simulink model "LQR_observer"  (R2022b)
settings: Solver=ode45  StartTime=0.0  StopTime=simulation_time  MaxStep=0.01  RelTol=1e-3  EnableMultiTasking=on
values from neighbouring files (symbols this model uses):
  AObs = [Phi - L*Cprime]    [ex2.m]
  BObs = [Gam L]    [ex2.m]
  C = eye(5)    [ex1.m]    (also in exercise2_LQRandObserver.m = Corig)
  CObs = eye(size(Phi))    [ex2.m]
  Cprim = [1 0 0 0 0 ... (first row only)    [ex2.m]
  DObs = zeros(size(Phi,1), size(L,2) + size(Gam,2))    [ex2.m]
  parameters = sol1.getSystemParameters    [exercise2_LQRandObserver.m]
  path_to_track =     [path_4.mat]
  sampling_time = 0.01    [exercise2_LQRandObserver.m]
  x0 = {x0_experiment_1}    [ex1.m]
  x0Obs = [0.01, 0, -0.02, 0, 0]    [ex2.m]
undefined symbols (not defined in the file or in its folder): lqr_gain, LQR_input_signal_ID
settings Model: Creator=ezequiel  LastModifiedBy=bapti
settings SolverCC: AlgebraicLoopSolver=TrustRegion
settings DataIOCC: ReturnWorkspaceOutputs=off
settings OptimizationCC: LifeSpan=inf
settings DebuggingCC: UnconnectedInputMsg=warning  UnconnectedOutputMsg=warning  UnconnectedLineMsg=warning  AllowSymbolicDim=off  PregeneratedLibrarySubsystemCodeDiagnostic=none  SFUnexpectedBacktrackingDiag=warning  SFNoUnconditionalDefaultTransitionDiag=warning  SFExecutionAtInitializationDiag=none  SFMachineParentedDataDiag=warning  ArithmeticOperatorsInVariantConditions=warning
settings ModelReferenceCC: EnableRefExpFcnMdlSchedulingChecks=on  PropagateSignalLabelsOutOfModel=off
settings SFSimCC: SimUseLocalCustomCode=off  CustomCodeUndefinedFunction=UseInterfaceOnly
settings RTWCC: RTWUseLocalCustomCode=off
settings CodeAppCC: StateflowObjectComments=on
settings GRTTargetCC: TargetLangStandard=C89/C90 (ANSI)
settings ConfigComp: CovMetricSettings=dw  CovSaveCumulativeToWorkspaceVar=on  CovSaveSingleToWorkspaceVar=on  CovExternalEMLEnable=off

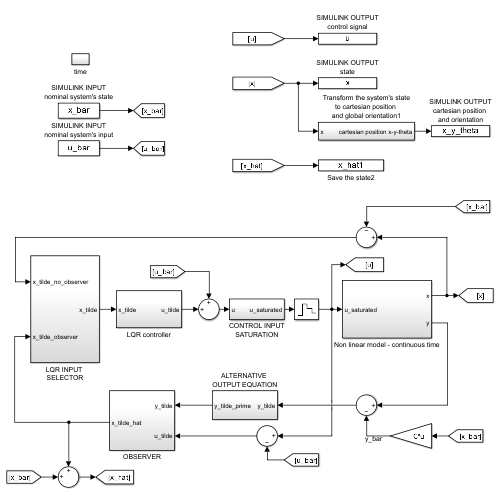
[thumbnail: Simulink's stored preview of the top-level diagram]
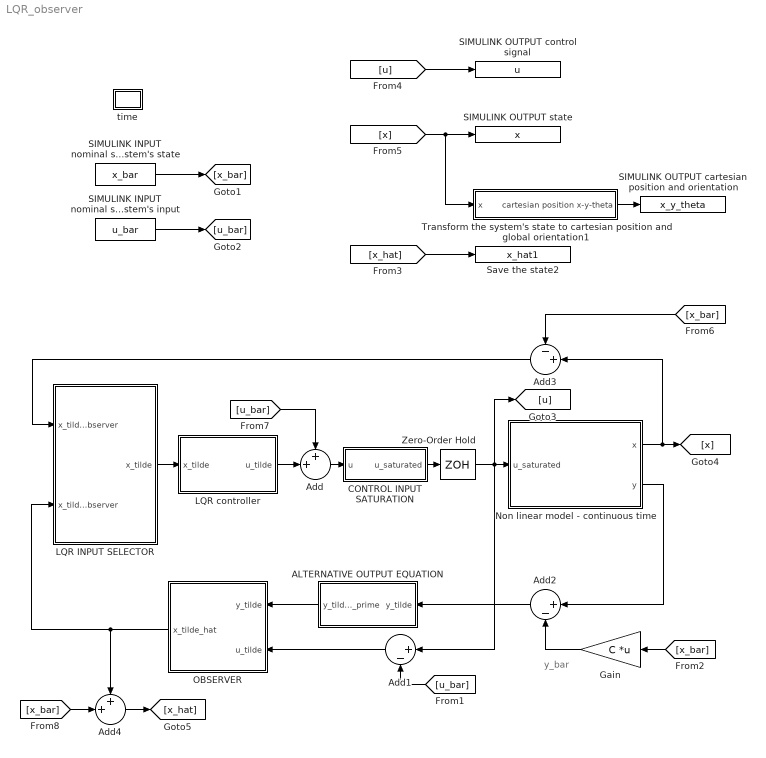
== system LQR_observer ==
  note: y_bar
  ALTERNATIVE OUTPUT EQUATION : Subsystem
  Add : Sum  Inputs=++|
  Add1 : Sum  Inputs=|+-
  Add2 : Sum  Inputs=|+-
  Add3 : Sum  Inputs=-+|
  Add4 : Sum  Inputs=++|
  CONTROL INPUT SATURATION : Subsystem
  Gain : Gain  Gain=C  Multiplication=Matrix(K*u)
  LQR INPUT SELECTOR : Subsystem
  LQR controller : Subsystem
  Non linear model - continuous time : Subsystem
  OBSERVER : Subsystem
  SIMULINK INPUT nominal system's input : FromWorkspace  VariableName=u_bar  SampleTime=sampling_time  OutputAfterFinalValue=Holding final value
  SIMULINK INPUT nominal system's state : FromWorkspace  VariableName=x_bar  SampleTime=sampling_time  OutputAfterFinalValue=Holding final value
  SIMULINK OUTPUT cartesian position and orientation : ToWorkspace  VariableName=x_y_theta  SampleTime=-1
  SIMULINK OUTPUT control signal : ToWorkspace  VariableName=u  SampleTime=-1
  SIMULINK OUTPUT state : ToWorkspace  VariableName=x  SampleTime=-1
  Save the state2 : ToWorkspace  VariableName=x_hat1  SampleTime=-1
  Transform the system's state to cartesian position and global orientation1 : Subsystem
  Zero-Order Hold : ZeroOrderHold  SampleTime=sampling_time
  time : Subsystem
  wires:
  SIMULINK INPUT nominal system's state/1 -> [x_bar]
  SIMULINK INPUT nominal system's input/1 -> [u_bar]
  [u] -> SIMULINK OUTPUT control signal/1
  [x] -> Transform the system's state to cartesian position and global orientation1/1(x), SIMULINK OUTPUT state/1
  Transform the system's state to cartesian position and global orientation1/1(cartesian position x-y-theta) -> SIMULINK OUTPUT cartesian position and orientation/1
  LQR INPUT SELECTOR/1(x_tilde) -> LQR controller/1(x_tilde)
  LQR controller/1(u_tilde) -> Add/2
  Add/1 -> CONTROL INPUT SATURATION/1(u)
  [u_bar] -> Add/1
  ALTERNATIVE OUTPUT EQUATION/1(y_tilde_prime) -> OBSERVER/1(y_tilde)
  OBSERVER/1(x_tilde_hat) -> LQR INPUT SELECTOR/2(x_tilde_observer), Add4/1
  [u_bar] -> Add1/2
  Add1/1 -> OBSERVER/2(u_tilde)
  [x_bar] -> Gain/1
  Gain/1 -> Add2/2
  Non linear model - continuous time/2(y) -> Add2/1
  Add2/1 -> ALTERNATIVE OUTPUT EQUATION/1(y_tilde)
  Non linear model - continuous time/1(x) -> [x], Add3/2
  Add3/1 -> LQR INPUT SELECTOR/1("x_tilde_no_observer ")
  [x_hat] -> Save the state2/1
  [x_bar] -> Add4/2
  Add4/1 -> [x_hat]
  [x_bar] -> Add3/1
  CONTROL INPUT SATURATION/1(u_saturated) -> Zero-Order Hold/1
  Zero-Order Hold/1 -> Add1/1, [u], Non linear model - continuous time/1(u_saturated)

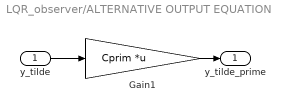
== system LQR_observer/ALTERNATIVE OUTPUT EQUATION ==
  y_tilde : Inport
  Gain1 : Gain  Gain=Cprim  Multiplication=Matrix(K*u)
  y_tilde_prime : Outport  VectorParamsAs1DForOutWhenUnconnected=off
  wires:
  Gain1/1 -> y_tilde_prime/1
  y_tilde/1 -> Gain1/1

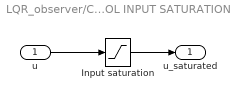
== system LQR_observer/CONTROL INPUT SATURATION ==
  u : Inport
  Input saturation : Saturate  UpperLimit=[Inf;4*pi]  LowerLimit=[0;-4*pi]
  u_saturated : Outport  VectorParamsAs1DForOutWhenUnconnected=off
  wires:
  u/1 -> Input saturation/1
  Input saturation/1 -> u_saturated/1

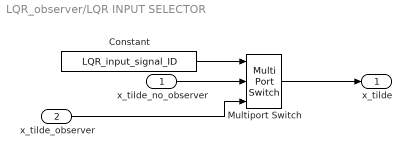
== system LQR_observer/LQR INPUT SELECTOR ==
  "x_tilde_no_observer " : Inport  PortDimensions=5
  x_tilde_observer : Inport  Port=2  PortDimensions=5
  Constant : Constant  Value=LQR_input_signal_ID
  Multiport Switch : MultiPortSwitch  Inputs=2  SaturateOnIntegerOverflow=off  InputSameDT=off
  x_tilde : Outport  VectorParamsAs1DForOutWhenUnconnected=off
  wires:
  "x_tilde_no_observer "/1 -> Multiport Switch/2
  x_tilde_observer/1 -> Multiport Switch/3
  Constant/1 -> Multiport Switch/1
  Multiport Switch/1 -> x_tilde/1

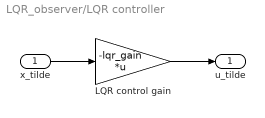
== system LQR_observer/LQR controller ==
  x_tilde : Inport  PortDimensions=5
  LQR control gain : Gain  Gain=-lqr_gain  Multiplication=Matrix(K*u)
  u_tilde : Outport  VectorParamsAs1DForOutWhenUnconnected=off
  wires:
  x_tilde/1 -> LQR control gain/1
  LQR control gain/1 -> u_tilde/1

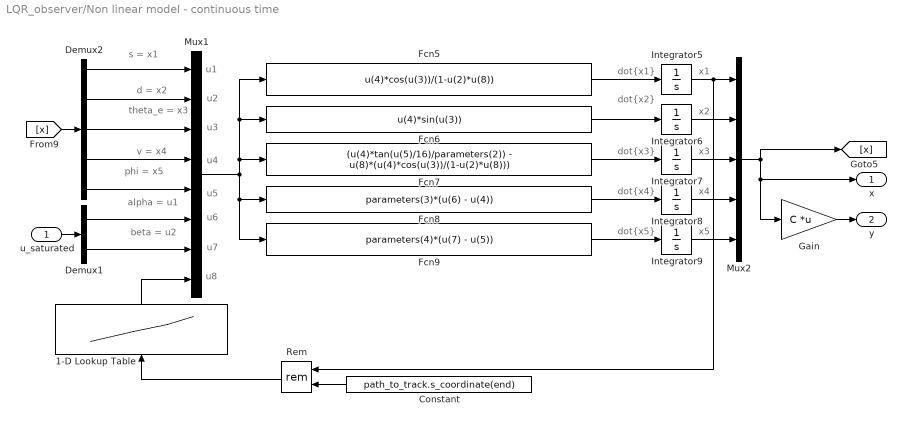
== system LQR_observer/Non linear model - continuous time ==
  note: s = x1
  note: dot{x1}
  note: d = x2
  note: theta_e = x3
  note: v = x4
  note: phi = x5
  note: alpha = u1
  note: beta = u2
  note: u1
  note: u2
  note: u3
  note: u4
  note: u5
  note: u6
  note: u7
  note: x1
  note: dot{x2}
  note: x2
  note: dot{x3}
  note: x3
  note: dot{x4}
  note: x4
  note: dot{x5}
  note: x5
  note: u8
  u_saturated : Inport
  1-D Lookup Table : Lookup_n-D  NumberOfTableDimensions=1  BreakpointsForDimension1=path_to_track.s_coordinate  Table=path_to_track.curvature  InternalRulePriority=Speed  RndMeth=Simplest
  Constant : Constant  Value=path_to_track.s_coordinate(end)
  Demux1 : Demux  Outputs=2
  Demux2 : Demux  Outputs=5
  Fcn5 : Fcn  Expr=u(4)*cos(u(3))/(1-u(2)*u(8))
  Fcn6 : Fcn  Expr=u(4)*sin(u(3))
  Fcn7 : Fcn  Expr=(u(4)*tan(u(5)/16)/parameters(2)) - u(8)*(u(4)*cos(u(3))/(1-u(2)*u(8)))
  Fcn8 : Fcn  Expr=parameters(3)*(u(6) - u(4))
  Fcn9 : Fcn  Expr=parameters(4)*(u(7) - u(5))
  Gain : Gain  Gain=C  Multiplication=Matrix(K*u)
  Integrator5 : Integrator  InitialCondition=x0(1)
  Integrator6 : Integrator  InitialCondition=x0(2)
  Integrator7 : Integrator  InitialCondition=x0(3)
  Integrator8 : Integrator  InitialCondition=x0(4)
  Integrator9 : Integrator  InitialCondition=x0(5)
  Mux1 : Mux  Inputs=8
  Mux2 : Mux  Inputs=5
  Rem : Math  Operator=rem  SignedPower=on
  x : Outport  VectorParamsAs1DForOutWhenUnconnected=off
  y : Outport  Port=2  VectorParamsAs1DForOutWhenUnconnected=off
  wires:
  u_saturated/1 -> Demux1/1
  Demux2/1 -> Mux1/1
  Demux2/2 -> Mux1/2
  Demux2/3 -> Mux1/3
  Demux2/4 -> Mux1/4
  Demux2/5 -> Mux1/5
  Demux1/1 -> Mux1/6
  Demux1/2 -> Mux1/7
  Integrator6/1 -> Mux2/2
  Integrator7/1 -> Mux2/3
  Integrator8/1 -> Mux2/4
  Integrator9/1 -> Mux2/5
  [x] -> Demux2/1
  1-D Lookup Table/1 -> Mux1/8
  Rem/1 -> 1-D Lookup Table/1
  Constant/1 -> Rem/2
  Integrator5/1 -> Rem/1, Mux2/1
  Mux2/1 -> Gain/1, x/1, [x]
  Gain/1 -> y/1
  Mux1/1 -> Fcn6/1, Fcn5/1, Fcn7/1, Fcn9/1, Fcn8/1
  Fcn8/1 -> Integrator8/1
  Fcn9/1 -> Integrator9/1
  Fcn7/1 -> Integrator7/1
  Fcn5/1 -> Integrator5/1
  Fcn6/1 -> Integrator6/1

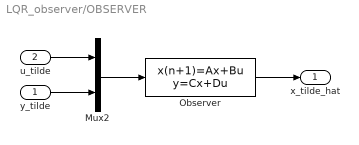
== system LQR_observer/OBSERVER ==
  y_tilde : Inport
  u_tilde : Inport  Port=2
  Mux2 : Mux  Inputs=2
  Observer : DiscreteStateSpace  A=AObs  B=BObs  C=CObs  D=DObs  InitialCondition=x0Obs  SampleTime=sampling_time
  x_tilde_hat : Outport  VectorParamsAs1DForOutWhenUnconnected=off
  wires:
  u_tilde/1 -> Mux2/1
  y_tilde/1 -> Mux2/2
  Mux2/1 -> Observer/1
  Observer/1 -> x_tilde_hat/1

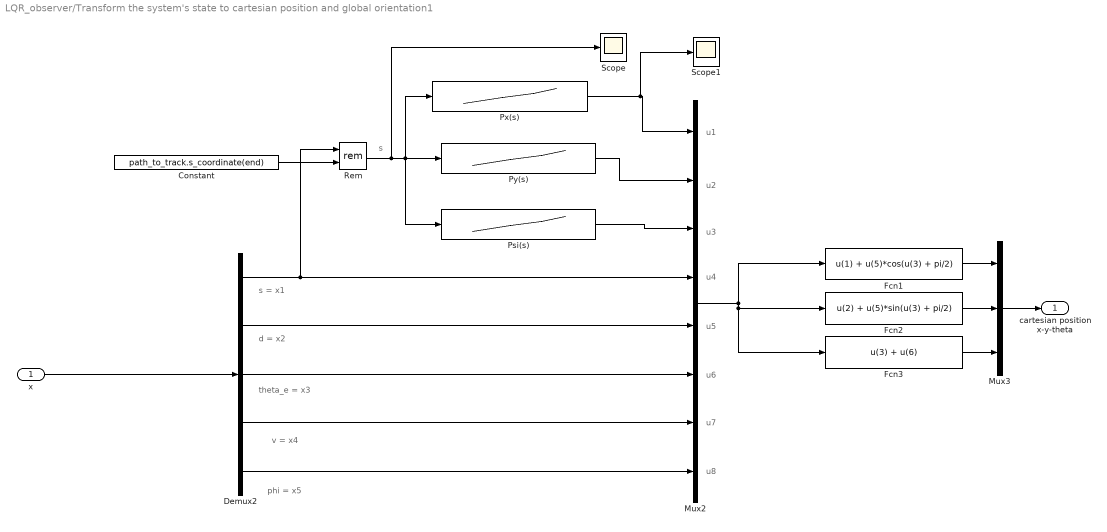
== system LQR_observer/Transform the system's state to cartesian position and global orientation1 ==
  note: s
  note: s = x1
  note: d = x2
  note: theta_e = x3
  note: v = x4
  note: phi = x5
  note: u1
  note: u2
  note: u3
  note: u4
  note: u5
  note: u6
  note: u7
  note: u8
  x : Inport
  Constant : Constant  Value=path_to_track.s_coordinate(end)
  Demux2 : Demux  Outputs=5
  Fcn1 : Fcn  Expr=u(1) + u(5)*cos(u(3) + pi/2)
  Fcn2 : Fcn  Expr=u(2) + u(5)*sin(u(3) + pi/2)
  Fcn3 : Fcn  Expr=u(3) + u(6)
  Mux2 : Mux  Inputs=8
  Mux3 : Mux  Inputs=3
  Psi(s) : Lookup_n-D  NumberOfTableDimensions=1  BreakpointsForDimension1=path_to_track.s_coordinate  Table=path_to_track.orientation  InternalRulePriority=Speed  RndMeth=Simplest
  Px(s) : Lookup_n-D  NumberOfTableDimensions=1  BreakpointsForDimension1=path_to_track.s_coordinate  Table=path_to_track.coordinates(:,1)  InternalRulePriority=Speed  RndMeth=Simplest
  Py(s) : Lookup_n-D  NumberOfTableDimensions=1  BreakpointsForDimension1=path_to_track.s_coordinate  Table=path_to_track.coordinates(:,2)  InternalRulePriority=Speed  RndMeth=Simplest
  Rem : Math  Operator=rem  SignedPower=on
  Scope : Scope
  Scope1 : Scope
  cartesian position x-y-theta : Outport  VectorParamsAs1DForOutWhenUnconnected=off
  wires:
  Demux2/1 -> Mux2/4, Rem/1
  Mux3/1 -> cartesian position x-y-theta/1
  x/1 -> Demux2/1
  Rem/1 -> Scope/1, Psi(s)/1, Px(s)/1, Py(s)/1
  Constant/1 -> Rem/2
  Px(s)/1 -> Scope1/1, Mux2/1
  Py(s)/1 -> Mux2/2
  Psi(s)/1 -> Mux2/3
  Mux2/1 -> Fcn3/1, Fcn2/1, Fcn1/1
  Fcn1/1 -> Mux3/1
  Fcn2/1 -> Mux3/2
  Fcn3/1 -> Mux3/3
  Demux2/2 -> Mux2/5
  Demux2/3 -> Mux2/6
  Demux2/4 -> Mux2/7
  Demux2/5 -> Mux2/8

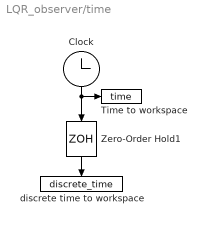
== system LQR_observer/time ==
  Clock : Clock
  Time to workspace : ToWorkspace  VariableName=time  SampleTime=-1
  Zero-Order Hold1 : ZeroOrderHold  SampleTime=sampling_time
  discrete time to workspace : ToWorkspace  VariableName=discrete_time  SampleTime=-1
  wires:
  Clock/1 -> Zero-Order Hold1/1, Time to workspace/1
  Zero-Order Hold1/1 -> discrete time to workspace/1
